simulink model "untitled4"  (R2022b)
settings: Solver=VariableStepAuto  StartTime=0.0  StopTime=10.0  RelTol=1e-3
settings Model: Creator=admin  LastModifiedBy=admin

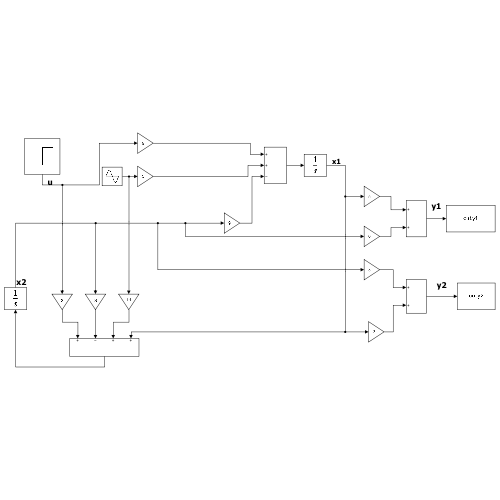
[thumbnail: Simulink's stored preview of the top-level diagram]
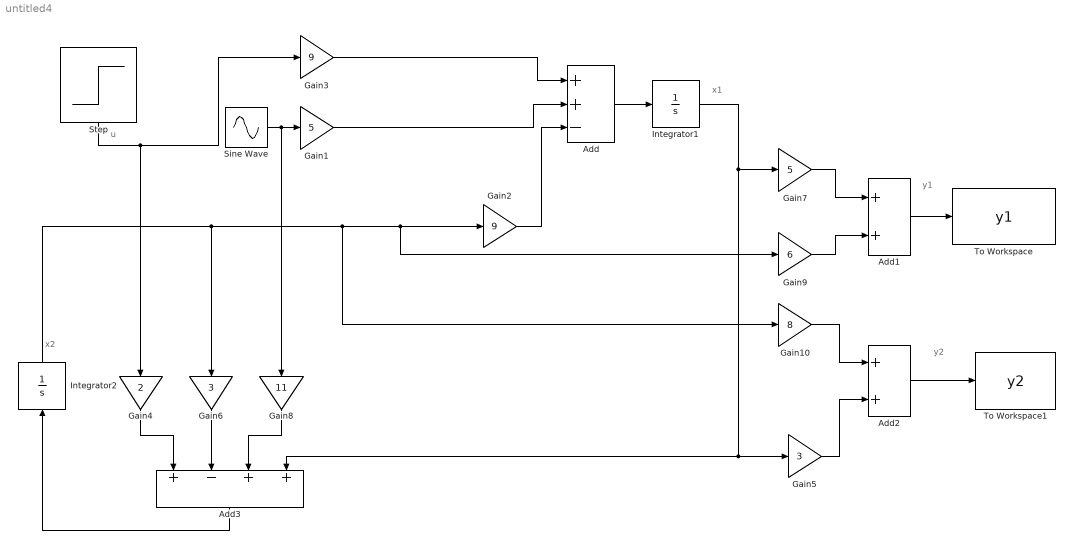
== system untitled4 ==
  note: u
  note: y2
  note: y1
  note: x1
  note: x2
  Add : Sum  Inputs=++-
  Add1 : Sum
  Add2 : Sum
  Add3 : Sum  Inputs=+-++
  Gain1 : Gain  Gain=5
  Gain10 : Gain  Gain=8
  Gain2 : Gain  Gain=9
  Gain3 : Gain  Gain=9
  Gain4 : Gain  Gain=2
  Gain5 : Gain  Gain=3
  Gain6 : Gain  Gain=3
  Gain7 : Gain  Gain=5
  Gain8 : Gain  Gain=11
  Gain9 : Gain  Gain=6
  Integrator1 : Integrator
  Integrator2 : Integrator
  Sine Wave : Sin  SampleTime=0
  Step : Step  SampleTime=0
  To Workspace : ToWorkspace  VariableName=y1  SaveFormat=Structure With Time  SampleTime=-1
  To Workspace1 : ToWorkspace  VariableName=y2  SaveFormat=Structure With Time  SampleTime=-1
  wires:
  Step/1 -> Gain3/1, Gain4/1
  Gain3/1 -> Add/1
  Gain1/1 -> Add/2
  Gain2/1 -> Add/3
  Add/1 -> Integrator1/1
  Sine Wave/1 -> Gain8/1, Gain1/1
  Integrator2/1 -> Gain6/1, Gain10/1, Gain9/1, Gain2/1
  Add3/1 -> Integrator2/1
  Gain4/1 -> Add3/1
  Gain6/1 -> Add3/2
  Gain8/1 -> Add3/3
  Integrator1/1 -> Gain5/1, Add3/4, Gain7/1
  Gain7/1 -> Add1/1
  Gain9/1 -> Add1/2
  Gain10/1 -> Add2/1
  Gain5/1 -> Add2/2
  Add1/1 -> To Workspace/1
  Add2/1 -> To Workspace1/1
